simulink model "Model_I7_Gust_Response_Time"  (Simulink 6.6)
settings: Solver=ode45  StartTime=tmin  StopTime=tmax  MaxStep=dt  RelTol=1e-3
values from neighbouring files (symbols this model uses):
  dt = 0.01    [Pgm_G11_Superposition.m]    (also in Pgm_G12_Num_Integration.m; Pgm_G13_Frequency_Domain.m = 0.0625; Pgm_H2_Response_Gusts_Control.m = 0.001; Pgm_H3_Ase_Gusts_Pid.m = 0.001)
  MC = inv(A)*C    [Pgm_H2_Response_Gusts_Control.m]    (also in Pgm_H3_Ase_Gusts_Pid.m; Pgm_I6_Dynamic_Manoeuvres.m = inv(M) * C; Pgm_I7_Gust_Time.m = MI * CC; Pgm_I91_Taxiing.m = inv(M) * CC)
  MFT = MI * FT    [Pgm_I7_Gust_Time.m]
  MFW = MI * FW    [Pgm_I7_Gust_Time.m]
  MK = inv(A)*K    [Pgm_H2_Response_Gusts_Control.m]    (also in Pgm_H3_Ase_Gusts_Pid.m; Pgm_I7_Gust_Time.m = MI * KK; Pgm_I91_Taxiing.m = inv(M) * K)
settings Model: Creator=Jan Wright  LastModifiedBy=Jan Wright
settings DataIOCC: SignalLoggingName=sigsOut
settings DebuggingCC: SignalResolutionControl=TryResolveAllWithWarning  SolverPrmCheckMsg=none  MultiTaskDSMMsg=warning  MultiTaskCondExecSysMsg=none  StrictBusMsg=None
settings HardwareCC: TargetUnknown=on
settings RTWCC: IncludeERTFirstTime=on
settings GRTTargetCC: ModelReferenceCompliant=off  MatFileLogging=off

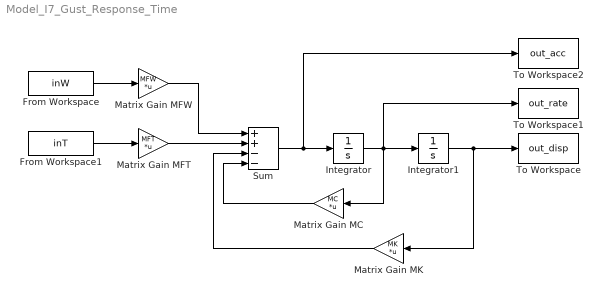
== system Model_I7_Gust_Response_Time ==
  From Workspace : FromWorkspace  VariableName=inW  SampleTime=dt
  From Workspace1 : FromWorkspace  VariableName=inT  SampleTime=dt
  Integrator : Integrator
  Integrator1 : Integrator
  Matrix Gain MC : Gain  Orientation=left  Gain=MC  Multiplication=Matrix(K*u)  SampleTime=dt  SaturateOnIntegerOverflow=on
  Matrix Gain MFT : Gain  Gain=MFT  Multiplication=Matrix(K*u)  SampleTime=dt  SaturateOnIntegerOverflow=on
  Matrix Gain MFW : Gain  Gain=MFW  Multiplication=Matrix(K*u)  SampleTime=dt  SaturateOnIntegerOverflow=on
  Matrix Gain MK : Gain  Orientation=left  Gain=MK  Multiplication=Matrix(K*u)  SampleTime=dt  SaturateOnIntegerOverflow=on
  Sum : Sum  Inputs=++--  SaturateOnIntegerOverflow=on
  To Workspace : ToWorkspace  VariableName=out_disp  SampleTime=dt  SaveFormat=Array
  To Workspace1 : ToWorkspace  VariableName=out_rate  SampleTime=dt  SaveFormat=Array
  To Workspace2 : ToWorkspace  VariableName=out_acc  SampleTime=dt  SaveFormat=Array
  wires:
  From Workspace/1 -> Matrix Gain MFW/1
  Matrix Gain MFW/1 -> Sum/1
  Sum/1 -> Integrator/1, To Workspace2/1
  Integrator/1 -> Matrix Gain MC/1, Integrator1/1, To Workspace1/1
  Integrator1/1 -> To Workspace/1, Matrix Gain MK/1
  Matrix Gain MC/1 -> Sum/4
  Matrix Gain MFT/1 -> Sum/2
  From Workspace1/1 -> Matrix Gain MFT/1
  Matrix Gain MK/1 -> Sum/3
